simulink model "UCT_KDeploy"  (R2025b)
settings: Solver=FixedStepDiscrete  StartTime=0.0  StopTime=inf  FixedStep=0.01  RelTol=1e-3  EnableMultiTasking=on
settings Model: STM32="{\"DigitalPortWrite\":[{\"ID\":\"newMicroMouseTemplate:84:3\"},{\"ID\":\"newMicroMouseTemplate:84:4\"},{\"ID\":\"newMicroMouseTemplate:84:5\"},{\"ID\":\"newMicroMouseTemplate:84:6\"},{\"ID\":\"newMicroMouseTemplate:84:7\"},{\"ID\":\"newMicroMouseTemplate:84:8\"},{\"ID\":\"newMicroMouseTemplate:84:9\"},{\"ID\":\"newMicroMouseTemplate:84:10\"},{\"ID\":\"MicroMouse_Deploy:84:3\"},{\"ID\":\"MicroMouse_Deploy:84:4\"},{\"ID\":\"MicroMouse_Deploy:84:5\"},{\"ID\":\"MicroMouse_Deploy:84:6\"},{\"ID\":\"MicroMouse_Deploy:84:7\"},{\"ID\":\"MicroMouse_Deploy:84:8\"},{\"ID\":\"MicroMouse_Deploy:84:9\"},{\"ID\":\"MicroMouse_Deploy:84:10\"}]}"  SimulationMode=external  ExtModeTrigDuration=10  Creator=JesseJabezArendse  LastModifiedBy=nicolls
settings SolverCC: AllowMultiTaskInputOutput=on  AutoInsertRateTranBlk=on  InsertRTBMode=Never (minimum delay)
settings OptimizationCC: DefaultUnderspecifiedDataType=single  EnhancedBackFolding=on  StrengthReduction=on  MemcpyThreshold=2048.0  PassReuseOutputArgsAs=Individual arguments  StateBitsets=on  DataBitsets=on  ZeroExternalMemoryAtStartup=off  ZeroInternalMemoryAtStartup=off  NoFixptDivByZeroProtection=on  MaxStackSize=4096  OptimizeBlockOrder=speed  DifferentSizesBufferReuse=on  MultiThreadedLoops=on  EfficientTunableParamExpr=on
settings DebuggingCC: MultiTaskCondExecSysMsg=none  ParameterOverflowMsg=none  ParameterPrecisionLossMsg=none  ParameterTunabilityLossMsg=error
settings HardwareCC: ProdBitPerPointer=32.0  ProdBitPerSizeT=32.0  ProdBitPerPtrDiffT=32.0  ProdLargestAtomicInteger=Long  ProdLargestAtomicFloat=Double  ProdWordSize=32.0  ProdLongLongMode=on  ProdHWDeviceType=ARM Compatible->ARM Cortex  TargetBitPerLong=64.0  TargetBitPerPointer=64.0  TargetBitPerSizeT=64.0  TargetBitPerPtrDiffT=64.0  TargetLongLongMode=on  TargetIntDivRoundTo=Zero  TargetEndianess=LittleEndian  TargetWordSize=64.0  TargetHWDeviceType=MATLAB Host
settings ModelReferenceCC: UpdateModelReferenceTargets=AssumeUpToDate  EnableParallelModelReferenceBuilds=on  ParallelModelReferenceMATLABWorkerInit=Copy Base Workspace  SupportModelReferenceSimTargetCustomCode=on
settings SFSimCC: SimCustomHeaderCode="#include \"simulink_wrapper.h\""  SimUserSources=../../src/kernel/src/simulink_wrapper.c  SimUserIncludeDirs=../../src/kernel/inc  MATLABDynamicMemAlloc=off  CustomCodeUndefinedFunction=DoNotDetect  SimHardwareAcceleration=native
settings RTWCC: SystemTargetFile=ert.tlc  TLCOptions=-p0  GenCodeOnly=on  TemplateMakefile=ert_default_tmf  RetainRTWFile=on  CustomHeaderCode="#include \"simulink_wrapper.h\""  CustomInclude=../../src/kernel/inc  Toolchain=GNU Tools for ARM Embedded Processors  BuildConfiguration=Specify  IncludeHyperlinkInReport=on  CodeExecutionProfiling=on  CodeProfilingInstrumentation=coarse  GPUComputeCapability=3.5  Description=Embedded Coder
settings CodeAppCC: ForceParamTrailComments=on  IgnoreCustomStorageClasses=off  OperatorAnnotations=on  SimulinkDataObjDesc=on  SFDataObjDesc=on  InsertBlockDesc=on
settings ERTTargetCC: ExtModeTransport=3.0  ExtModeStaticAlloc=on  ExtModeStaticAllocSize=2048.0  ExtModeMexFile=ext_xcp  ExtModeIntrfLevel=Level2 - Open  InlinedParameterPlacement=Hierarchical  ERTCustomFileTemplate=example_file_process.tlc  DynamicArrayContainerType=coder::array  TargetLangStandard=C99 (ISO)  CodeReplacementLibrary=ARM Cortex-M  SupportNonFinite=off  SupportComplex=off

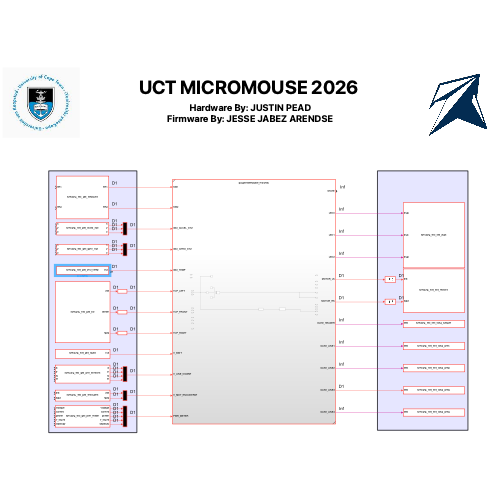
[thumbnail: Simulink's stored preview of the top-level diagram]
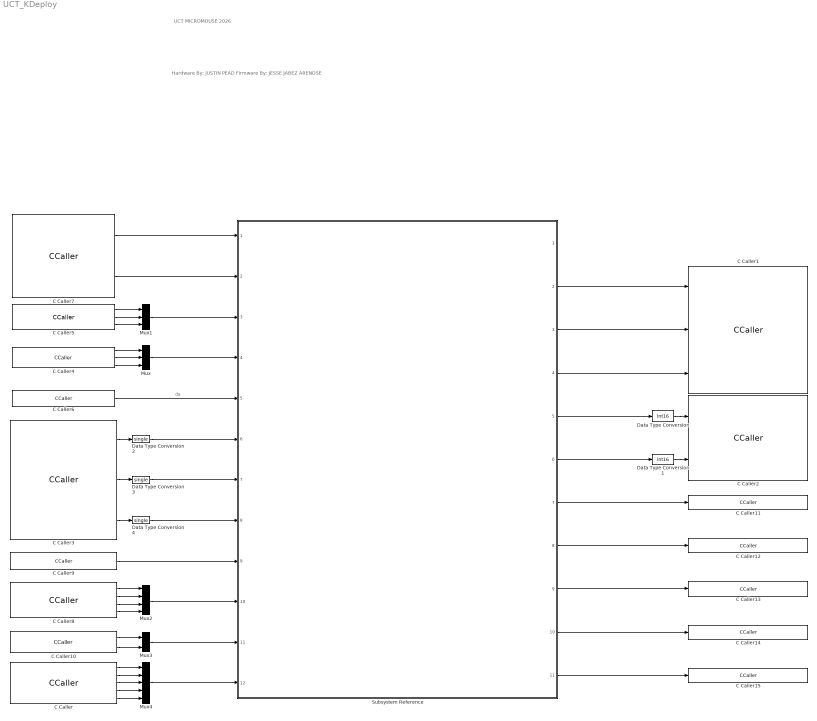
== system UCT_KDeploy ==
  note: UCT MICROMOUSE 2026
  note: Hardware By: JUSTIN PEAD
      | Firmware By: JESSE JABEZ ARENDSE
  C Caller : CCaller  FunctionName=simulink_ext_get_pwr_meter  PortSpecificationStruct="%)30     .    $ D   8    (     @         %    \"     4    !     0         %  0 \"0    $    _    07)G3F%M90  4&]R=$YA;64 4V-O<&4     26YD97@     5'EP90      4VEZ90      27-';&]B86P   X    X    !@    @    $          4    (     0    <    !         !     '    =F]L=&%G90 .    .     8    (    !          %    \"     $    '     0         0    !P   '9O;'1A9V4 #@   $     &    \"     0         !0    @    !   ...(+2748 chars)"
  C Caller1 : CCaller  FunctionName=simulink_ext_set_leds  PortSpecificationStruct="%)30     .    6 4   8    (     @         %    \"     ,    !     0         %  0 \"0    $    _    07)G3F%M90  4&]R=$YA;64 4V-O<&4     26YD97@     5'EP90      4VEZ90      27-';&]B86P   X    P    !@    @    $          4    (     0    0    !         !  ! !L960P#@   #     &    \"     0         !0    @    !    !     $         $  $ &QE9# .    .     8    (    !          %    \"     $    %     0         0    !0   $EN<'5T    #@   #@    &    \"     8         !0    @    !     0    $         \"0    @               X    X    !@    @    $          4    (     0    4    !         !     %    =6EN=#@    .    ,     8    (    !          %    \"     $    !     0         0  $ ,0    X    P    !@    @    ) @        4    (     0    $    !          (  0      #@   #     &    \"     0         !0    @    !    !     $         $  $ &QE9#$.    ,     8    (    !          %    \"     $    $     0         0  0 ;&5D,0X    X    !@    @    $          4    (     0    4    !         !     %    26YP=70    .    .     8    (    !@         %    \"     $    !     0         )    \"            / _#@   #@    &    \"     0         !0    @    !    !0    $         $     4   !U:6YT.     X    P    !@    @    $          4    (     0    $    !         !   0 Q    #@   #     &    \"     D\"        !0    @    !     0    $          @ !       .    ,     8    (    !          %    \"     $    $     0         0  0 ;&5D,@X    P    !@    @    $          4    (     0    0    !         !  ! !L960R#@   #@    &    \"     0         !0    @    !    !0    $         $     4   !);G!U=     X    X    !@    @    &          4    (     0    $    !          D    (             $ .    .     8    (    !          %    \"     $    %     0         0    !0   '5I;G0X    #@   #     &    \"     0         !0    @    !     0    $         $  ! #$    .    ,     8    (    \"0(        %    \"     $    !     0         \"  $"
  C Caller10 : CCaller  FunctionName=simulink_ext_get_encoders  PortSpecificationStruct="%)30     .    V ,   8    (     @         %    \"     (    !     0         %  0 \"0    $    _    07)G3F%M90  4&]R=$YA;64 4V-O<&4     26YD97@     5'EP90      4VEZ90      27-';&]B86P   X    P    !@    @    $          4    (     0    0    !         !  ! !L969T#@   #     &    \"     0         !0    @    !    !     $         $  $ &QE9G0.    0     8    (    !          %    \"     $    +     0         0    \"P   $EN<'5T3W5T<'5T       .    .     8    (    !@         %    \"     $    !     0         )    \"               #@   #@    &    \"     0         !0    @    !    !0    $         $     4   !I;G0S,@    X    P    !@    @    $          4    (     0    (    !         !   @ M,0  #@   #     &    \"     D\"        !0    @    !     0    $          @ !       .    .     8    (    !          %    \"     $    %     0         0    !0   ')I9VAT    #@   #@    &    \"     0         !0    @    !    !0    $         $     4   !R:6=H=     X   !     !@    @    $          4    (     0    L    !         !     +    26YP=71/=71P=70       X    X    !@    @    &          4    (     0    $    !          D    (            \\#\\.    .     8    (    !          %    \"     $    %     0         0    !0   &EN=#,R    #@   #     &    \"     0         !0    @    !     @    $         $  \" \"TQ   .    ,     8    (    \"0(        %    \"     $    !     0         \"  $"
  C Caller11 : CCaller  FunctionName=simulink_ext_set_oled_header  PortSpecificationStruct="%)30     .    & (   8    (     @         %    \"     $    !     0         %  0 \"0    $    _    07)G3F%M90  4&]R=$YA;64 4V-O<&4     26YD97@     5'EP90      4VEZ90      27-';&]B86P   X    P    !@    @    $          4    (     0    0    !         !  ! !T97AT#@   #     &    \"     0         !0    @    !    !     $         $  $ '1E>'0.    .     8    (    !          %    \"     $    %     0         0    !0   $EN<'5T    #@   #@    &    \"     8         !0    @    !     0    $         \"0    @               X    X    !@    @    $          4    (     0    8    !         !     &    <W1R:6YG   .    ,     8    (    !          %    \"     $    !     0         0  $ ,0    X    P    !@    @    ) @        4    (     0    $    !          (  0"
  C Caller12 : CCaller  FunctionName=simulink_ext_set_oled_line1  PortSpecificationStruct="%)30     .    & (   8    (     @         %    \"     $    !     0         %  0 \"0    $    _    07)G3F%M90  4&]R=$YA;64 4V-O<&4     26YD97@     5'EP90      4VEZ90      27-';&]B86P   X    P    !@    @    $          4    (     0    0    !         !  ! !T97AT#@   #     &    \"     0         !0    @    !    !     $         $  $ '1E>'0.    .     8    (    !          %    \"     $    %     0         0    !0   $EN<'5T    #@   #@    &    \"     8         !0    @    !     0    $         \"0    @               X    X    !@    @    $          4    (     0    8    !         !     &    <W1R:6YG   .    ,     8    (    !          %    \"     $    !     0         0  $ ,0    X    P    !@    @    ) @        4    (     0    $    !          (  0"
  C Caller13 : CCaller  FunctionName=simulink_ext_set_oled_line2  PortSpecificationStruct="%)30     .    & (   8    (     @         %    \"     $    !     0         %  0 \"0    $    _    07)G3F%M90  4&]R=$YA;64 4V-O<&4     26YD97@     5'EP90      4VEZ90      27-';&]B86P   X    P    !@    @    $          4    (     0    0    !         !  ! !T97AT#@   #     &    \"     0         !0    @    !    !     $         $  $ '1E>'0.    .     8    (    !          %    \"     $    %     0         0    !0   $EN<'5T    #@   #@    &    \"     8         !0    @    !     0    $         \"0    @               X    X    !@    @    $          4    (     0    8    !         !     &    <W1R:6YG   .    ,     8    (    !          %    \"     $    !     0         0  $ ,0    X    P    !@    @    ) @        4    (     0    $    !          (  0"
  C Caller14 : CCaller  FunctionName=simulink_ext_set_oled_line3  PortSpecificationStruct="%)30     .    & (   8    (     @         %    \"     $    !     0         %  0 \"0    $    _    07)G3F%M90  4&]R=$YA;64 4V-O<&4     26YD97@     5'EP90      4VEZ90      27-';&]B86P   X    P    !@    @    $          4    (     0    0    !         !  ! !T97AT#@   #     &    \"     0         !0    @    !    !     $         $  $ '1E>'0.    .     8    (    !          %    \"     $    %     0         0    !0   $EN<'5T    #@   #@    &    \"     8         !0    @    !     0    $         \"0    @               X    X    !@    @    $          4    (     0    8    !         !     &    <W1R:6YG   .    ,     8    (    !          %    \"     $    !     0         0  $ ,0    X    P    !@    @    ) @        4    (     0    $    !          (  0"
  C Caller15 : CCaller  FunctionName=simulink_ext_set_oled_line4  PortSpecificationStruct="%)30     .    & (   8    (     @         %    \"     $    !     0         %  0 \"0    $    _    07)G3F%M90  4&]R=$YA;64 4V-O<&4     26YD97@     5'EP90      4VEZ90      27-';&]B86P   X    P    !@    @    $          4    (     0    0    !         !  ! !T97AT#@   #     &    \"     0         !0    @    !    !     $         $  $ '1E>'0.    .     8    (    !          %    \"     $    %     0         0    !0   $EN<'5T    #@   #@    &    \"     8         !0    @    !     0    $         \"0    @               X    X    !@    @    $          4    (     0    8    !         !     &    <W1R:6YG   .    ,     8    (    !          %    \"     $    !     0         0  $ ,0    X    P    !@    @    ) @        4    (     0    $    !          (  0"
  C Caller2 : CCaller  FunctionName=simulink_ext_set_motors  PortSpecificationStruct="%)30     .    R ,   8    (     @         %    \"     (    !     0         %  0 \"0    $    _    07)G3F%M90  4&]R=$YA;64 4V-O<&4     26YD97@     5'EP90      4VEZ90      27-';&]B86P   X    P    !@    @    $          4    (     0    0    !         !  ! !L969T#@   #     &    \"     0         !0    @    !    !     $         $  $ &QE9G0.    .     8    (    !          %    \"     $    %     0         0    !0   $EN<'5T    #@   #@    &    \"     8         !0    @    !     0    $         \"0    @               X    X    !@    @    $          4    (     0    4    !         !     %    :6YT,38    .    ,     8    (    !          %    \"     $    !     0         0  $ ,0    X    P    !@    @    ) @        4    (     0    $    !          (  0      #@   #@    &    \"     0         !0    @    !    !0    $         $     4   !R:6=H=     X    X    !@    @    $          4    (     0    4    !         !     %    <FEG:'0    .    .     8    (    !          %    \"     $    %     0         0    !0   $EN<'5T    #@   #@    &    \"     8         !0    @    !     0    $         \"0    @           #P/PX    X    !@    @    $          4    (     0    4    !         !     %    :6YT,38    .    ,     8    (    !          %    \"     $    !     0         0  $ ,0    X    P    !@    @    ) @        4    (     0    $    !          (  0"
  C Caller3 : CCaller  FunctionName=simulink_ext_get_tof  PortSpecificationStruct="%)30     .    > 4   8    (     @         %    \"     ,    !     0         %  0 \"0    $    _    07)G3F%M90  4&]R=$YA;64 4V-O<&4     26YD97@     5'EP90      4VEZ90      27-';&]B86P   X    P    !@    @    $          4    (     0    0    !         !  ! !L969T#@   #     &    \"     0         !0    @    !    !     $         $  $ &QE9G0.    .     8    (    !          %    \"     $    &     0         0    !@   $]U='!U=   #@   #@    &    \"     8         !0    @    !     0    $         \"0    @               X    X    !@    @    $          4    (     0    8    !         !     &    =6EN=#$V   .    ,     8    (    !          %    \"     $    \"     0         0  ( +3$   X    P    !@    @    ) @        4    (     0    $    !          (  0      #@   #@    &    \"     0         !0    @    !    !@    $         $     8   !C96YT97(   X    X    !@    @    $          4    (     0    8    !         !     &    8V5N=&5R   .    .     8    (    !          %    \"     $    &     0         0    !@   $]U='!U=   #@   #@    &    \"     8         !0    @    !     0    $         \"0    @           #P/PX    X    !@    @    $          4    (     0    8    !         !     &    =6EN=#$V   .    ,     8    (    !          %    \"     $    \"     0         0  ( +3$   X    P    !@    @    ) @        4    (     0    $    !          (  0      #@   #@    &    \"     0         !0    @    !    !0    $         $     4   !R:6=H=     X    X    !@    @    $          4    (     0    4    !         !     %    <FEG:'0    .    .     8    (    !          %    \"     $    &     0         0    !@   $]U='!U=   #@   #@    &    \"     8         !0    @    !     0    $         \"0    @             0 X    X    !@    @    $          4    (     0    8    !         !     &    =6EN=#$V   .    ,     8    (    !          %    \"     $    \"     0         0  ( +3$   X    P    !@    @    ) @        4    (     0    $    !          (  0"
  C Caller4 : CCaller  FunctionName=simulink_ext_get_gyro_xyz  PortSpecificationStruct="%)30     .    < 4   8    (     @         %    \"     ,    !     0         %  0 \"0    $    _    07)G3F%M90  4&]R=$YA;64 4V-O<&4     26YD97@     5'EP90      4VEZ90      27-';&]B86P   X    P    !@    @    $          4    (     0    $    !         !   0!X    #@   #     &    \"     0         !0    @    !     0    $         $  ! '@    .    0     8    (    !          %    \"     $    +     0         0    \"P   $EN<'5T3W5T<'5T       .    .     8    (    !@         %    \"     $    !     0         )    \"               #@   #@    &    \"     0         !0    @    !    !@    $         $     8   !S:6YG;&4   X    P    !@    @    $          4    (     0    (    !         !   @ M,0  #@   #     &    \"     D\"        !0    @    !     0    $          @ !       .    ,     8    (    !          %    \"     $    !     0         0  $ >0    X    P    !@    @    $          4    (     0    $    !         !   0!Y    #@   $     &    \"     0         !0    @    !    \"P    $         $     L   !);G!U=$]U='!U=       #@   #@    &    \"     8         !0    @    !     0    $         \"0    @           #P/PX    X    !@    @    $          4    (     0    8    !         !     &    <VEN9VQE   .    ,     8    (    !          %    \"     $    \"     0         0  ( +3$   X    P    !@    @    ) @        4    (     0    $    !          (  0      #@   #     &    \"     0         !0    @    !     0    $         $  ! 'H    .    ,     8    (    !          %    \"     $    !     0         0  $ >@    X   !     !@    @    $          4    (     0    L    !         !     +    26YP=71/=71P=70       X    X    !@    @    &          4    (     0    $    !          D    (             $ .    .     8    (    !          %    \"     $    &     0         0    !@   '-I;F=L90  #@   #     &    \"     0         !0    @    !     @    $         $  \" \"TQ   .    ,     8    (    \"0(        %    \"     $    !     0         \"  $"
  C Caller5 : CCaller  FunctionName=simulink_ext_get_accel_xyz  PortSpecificationStruct="%)30     .    < 4   8    (     @         %    \"     ,    !     0         %  0 \"0    $    _    07)G3F%M90  4&]R=$YA;64 4V-O<&4     26YD97@     5'EP90      4VEZ90      27-';&]B86P   X    P    !@    @    $          4    (     0    $    !         !   0!X    #@   #     &    \"     0         !0    @    !     0    $         $  ! '@    .    0     8    (    !          %    \"     $    +     0         0    \"P   $EN<'5T3W5T<'5T       .    .     8    (    !@         %    \"     $    !     0         )    \"               #@   #@    &    \"     0         !0    @    !    !@    $         $     8   !S:6YG;&4   X    P    !@    @    $          4    (     0    (    !         !   @ M,0  #@   #     &    \"     D\"        !0    @    !     0    $          @ !       .    ,     8    (    !          %    \"     $    !     0         0  $ >0    X    P    !@    @    $          4    (     0    $    !         !   0!Y    #@   $     &    \"     0         !0    @    !    \"P    $         $     L   !);G!U=$]U='!U=       #@   #@    &    \"     8         !0    @    !     0    $         \"0    @           #P/PX    X    !@    @    $          4    (     0    8    !         !     &    <VEN9VQE   .    ,     8    (    !          %    \"     $    \"     0         0  ( +3$   X    P    !@    @    ) @        4    (     0    $    !          (  0      #@   #     &    \"     0         !0    @    !     0    $         $  ! 'H    .    ,     8    (    !          %    \"     $    !     0         0  $ >@    X   !     !@    @    $          4    (     0    L    !         !     +    26YP=71/=71P=70       X    X    !@    @    &          4    (     0    $    !          D    (             $ .    .     8    (    !          %    \"     $    &     0         0    !@   '-I;F=L90  #@   #     &    \"     0         !0    @    !     @    $         $  \" \"TQ   .    ,     8    (    \"0(        %    \"     $    !     0         \"  $"
  C Caller6 : CCaller  FunctionName=simulink_ext_get_imu_temp  PortSpecificationStruct="%)30     .    & (   8    (     @         %    \"     $    !     0         %  0 \"0    $    _    07)G3F%M90  4&]R=$YA;64 4V-O<&4     26YD97@     5'EP90      4VEZ90      27-';&]B86P   X    P    !@    @    $          4    (     0    ,    !         !   P!O=70 #@   #     &    \"     0         !0    @    !     P    $         $  # &]U=  .    .     8    (    !          %    \"     $    &     0         0    !@   $]U='!U=   #@   #@    &    \"     8         !0    @    !     0    $         \"0    @               X    X    !@    @    $          4    (     0    8    !         !     &    <VEN9VQE   .    ,     8    (    !          %    \"     $    !     0         0  $ ,0    X    P    !@    @    ) @        4    (     0    $    !          (  0"
  C Caller7 : CCaller  FunctionName=simulink_ext_get_switches  PortSpecificationStruct="%)30     .    R ,   8    (     @         %    \"     (    !     0         %  0 \"0    $    _    07)G3F%M90  4&]R=$YA;64 4V-O<&4     26YD97@     5'EP90      4VEZ90      27-';&]B86P   X    P    !@    @    $          4    (     0    ,    !         !   P!S=S$ #@   #     &    \"     0         !0    @    !     P    $         $  # '-W,0 .    0     8    (    !          %    \"     $    +     0         0    \"P   $EN<'5T3W5T<'5T       .    .     8    (    !@         %    \"     $    !     0         )    \"               #@   #@    &    \"     0         !0    @    !    !0    $         $     4   !U:6YT.     X    P    !@    @    $          4    (     0    (    !         !   @ M,0  #@   #     &    \"     D\"        !0    @    !     0    $          @ !       .    ,     8    (    !          %    \"     $    #     0         0  , <W<R  X    P    !@    @    $          4    (     0    ,    !         !   P!S=S( #@   $     &    \"     0         !0    @    !    \"P    $         $     L   !);G!U=$]U='!U=       #@   #@    &    \"     8         !0    @    !     0    $         \"0    @           #P/PX    X    !@    @    $          4    (     0    4    !         !     %    =6EN=#@    .    ,     8    (    !          %    \"     $    \"     0         0  ( +3$   X    P    !@    @    ) @        4    (     0    $    !          (  0"
  C Caller8 : CCaller  FunctionName=simulink_ext_get_line_sensors  PortSpecificationStruct="%)30     .    & <   8    (     @         %    \"     0    !     0         %  0 \"0    $    _    07)G3F%M90  4&]R=$YA;64 4V-O<&4     26YD97@     5'EP90      4VEZ90      27-';&]B86P   X    P    !@    @    $          4    (     0    (    !         !   @!F;   #@   #     &    \"     0         !0    @    !     @    $         $  \" &9L   .    0     8    (    !          %    \"     $    +     0         0  ...(+2073 chars)"
  C Caller9 : CCaller  FunctionName=simulink_ext_get_vbatt  PortSpecificationStruct="%)30     .    & (   8    (     @         %    \"     $    !     0         %  0 \"0    $    _    07)G3F%M90  4&]R=$YA;64 4V-O<&4     26YD97@     5'EP90      4VEZ90      27-';&]B86P   X    P    !@    @    $          4    (     0    ,    !         !   P!O=70 #@   #     &    \"     0         !0    @    !     P    $         $  # &]U=  .    .     8    (    !          %    \"     $    &     0         0    !@   $]U='!U=   #@   #@    &    \"     8         !0    @    !     0    $         \"0    @               X    X    !@    @    $          4    (     0    8    !         !     &    <VEN9VQE   .    ,     8    (    !          %    \"     $    !     0         0  $ ,0    X    P    !@    @    ) @        4    (     0    $    !          (  0"
  Data Type Conversion : DataTypeConversion  OutDataTypeStr=int16  SaturateOnIntegerOverflow=off  RndMeth=Floor
  Data Type Conversion1 : DataTypeConversion  OutDataTypeStr=int16  SaturateOnIntegerOverflow=off  RndMeth=Floor
  Data Type Conversion2 : DataTypeConversion  OutDataTypeStr=single  SaturateOnIntegerOverflow=off  RndMeth=Floor
  Data Type Conversion3 : DataTypeConversion  OutDataTypeStr=single  SaturateOnIntegerOverflow=off  RndMeth=Floor
  Data Type Conversion4 : DataTypeConversion  OutDataTypeStr=single  SaturateOnIntegerOverflow=off  RndMeth=Floor
  Mux : Mux  Inputs=3
  Mux1 : Mux  Inputs=3
  Mux2 : Mux
  Mux3 : Mux  Inputs=2
  Mux4 : Mux  Inputs=5
  Subsystem Reference : Subsystem  ReferencedSubsystem=StudentTemplate_minimal
  wires:
  Subsystem Reference/6 -> Data Type Conversion1/1
  Subsystem Reference/5 -> Data Type Conversion/1
  C Caller3/1 -> Data Type Conversion2/1
  C Caller3/2 -> Data Type Conversion3/1
  C Caller3/3 -> Data Type Conversion4/1
  C Caller4/1 -> Mux/1
  C Caller4/2 -> Mux/2
  C Caller4/3 -> Mux/3
  Mux/1 -> Subsystem Reference/4
  C Caller5/1 -> Mux1/1
  C Caller5/2 -> Mux1/2
  C Caller5/3 -> Mux1/3
  Data Type Conversion/1 -> C Caller2/1
  Data Type Conversion1/1 -> C Caller2/2
  C Caller7/1 -> Subsystem Reference/1
  C Caller7/2 -> Subsystem Reference/2
  Data Type Conversion2/1 -> Subsystem Reference/6
  Data Type Conversion3/1 -> Subsystem Reference/7
  Data Type Conversion4/1 -> Subsystem Reference/8
  C Caller6/1 -> Subsystem Reference/5  "da"
  Mux1/1 -> Subsystem Reference/3
  C Caller8/1 -> Mux2/1
  C Caller8/2 -> Mux2/2
  C Caller8/3 -> Mux2/3
  C Caller8/4 -> Mux2/4
  Mux2/1 -> Subsystem Reference/10
  C Caller9/1 -> Subsystem Reference/9
  C Caller10/1 -> Mux3/1
  C Caller10/2 -> Mux3/2
  Mux3/1 -> Subsystem Reference/11
  C Caller/5 -> Mux4/5
  C Caller/4 -> Mux4/4
  C Caller/3 -> Mux4/3
  C Caller/2 -> Mux4/2
  C Caller/1 -> Mux4/1
  Mux4/1 -> Subsystem Reference/12
  Subsystem Reference/2 -> C Caller1/1
  Subsystem Reference/3 -> C Caller1/2
  Subsystem Reference/4 -> C Caller1/3
  Subsystem Reference/11 -> C Caller15/1
  Subsystem Reference/10 -> C Caller14/1
  Subsystem Reference/9 -> C Caller13/1
  Subsystem Reference/8 -> C Caller12/1
  Subsystem Reference/7 -> C Caller11/1
